simulink model "final_hybrid_system_load_variation"  (R2018a)
settings: Solver=ode23tb  StartTime=0.0  StopTime=4  FixedStep=1e-6  RelTol=1e-3
values from neighbouring files (symbols this model uses):
  Dp = 636    [sychrocovnverter.m]
  Dq = 100/155.35    (= 0.643707756678)    [sychrocovnverter.m]
  J = 2    [sychrocovnverter.m]
  K = 500    [sychrocovnverter.m]
  p = 1    [sychrocovnverter.m]
  Ts = 1e-6    (= 1e-06)    [sychrocovnverter.m]
  w_n = 2*pi*50    (= 314.159265359)    [sychrocovnverter.m]
  w_ref = w_n    (= 314.159265359)    [sychrocovnverter.m]
undefined symbols (not defined in the file or in its folder): sigbuilder_block
libraries: powerlib x73, powerlib_meascontrol x12, simulink x3, sps_avr x1, spsHTGModel x1, re_lib x1
settings Model: SimulationMode=accelerator  Creator=deep  LastModifiedBy=Electrical
settings SolverCC: AlgebraicLoopSolver=LineSearch
settings OptimizationCC: EfficientMapNaN2IntZero=off
settings HardwareCC: TargetBitPerPointer=64  TargetBitPerSizeT=64  TargetBitPerPtrDiffT=64  TargetLongLongMode=on  TargetIntDivRoundTo=Zero  TargetEndianess=LittleEndian  TargetWordSize=64  TargetHWDeviceType=MATLAB Host  ProdEqTarget=off
settings SFSimCC: SimUseLocalCustomCode=on
settings RTWCC: RTWUseLocalCustomCode=on
settings CodeAppCC: MaxIdLength=128
settings GRTTargetCC: TargetLangStandard=C89/C90 (ANSI)  CombineOutputUpdateFcns=off  GRTInterface=on

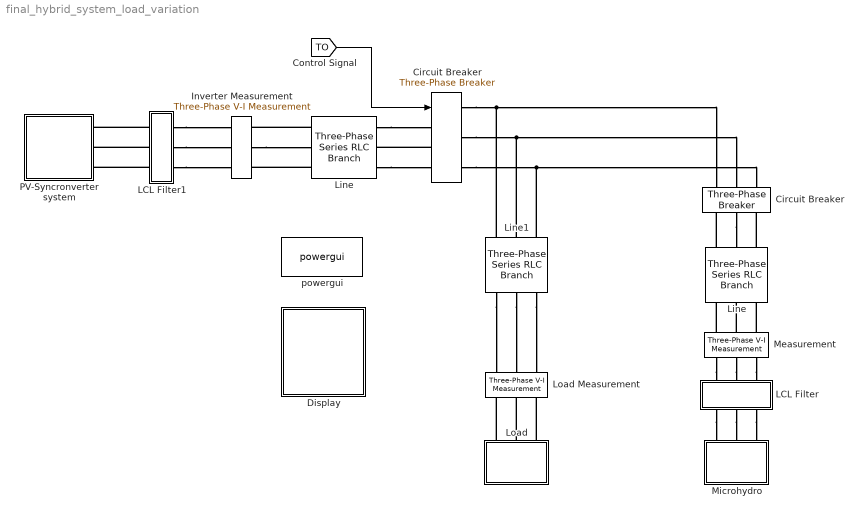
== system final_hybrid_system_load_variation ==
  Circuit Breaker : powerlib/Elements/Three-Phase Breaker  InitialState=open  SwitchA=on  SwitchB=on  SwitchC=on  SwitchTimes=[0.5 4]  External=off  BreakerResistance=0.00001  SnubberResistance=500000  SnubberCapacitance=inf  Measurements=None
  "Circuit Breaker  " : powerlib/Elements/Three-Phase Breaker  InitialState=closed  SwitchA=on  SwitchB=on  SwitchC=on  SwitchTimes=[0.5 4]  External=on  BreakerResistance=0.00001  SnubberResistance=500000  SnubberCapacitance=inf  Measurements=None
  Display : Subsystem
  Inverter Measurement : powerlib/Measurements/Three-Phase V-I Measurement  VoltageMeasurement=phase-to-ground  SetLabelV=on  LabelV=Vinv  Vpu=off  VpuLL=off  CurrentMeasurement=yes  SetLabelI=on  LabelI=Iinv  Ipu=off  Pbase=100e6  Vbase=500e3  OutputType=Complex  PhasorSimulation=off  PSBequivalent=0
  LCL Filter : Subsystem  mask{L=0.5e-3, C=100e-6}
      mask prompts: L "Inductance(L)"; C "Capacitance(C)"
  LCL Filter1 : Subsystem  mask{L=10e-3, C=0.5e-6}
      mask prompts: L "Inductance(L)"; C "Capacitance(C)"
  Line : powerlib/Elements/Three-Phase Series RLC Branch  LConnTagsString=A|B|C  RConnTagsString=A|B|C  BranchType=RL  Resistance=0.1  Inductance=0.0125  Capacitance=0  Measurements=None
  "Line  " : powerlib/Elements/Three-Phase Series RLC Branch  LConnTagsString=A|B|C  RConnTagsString=A|B|C  BranchType=RL  Resistance=0.1  Inductance=0.0125  Capacitance=0  Measurements=None
  Line1 : powerlib/Elements/Three-Phase Series RLC Branch  LConnTagsString=A|B|C  RConnTagsString=A|B|C  BranchType=RL  Resistance=0.1  Inductance=0.005  Capacitance=0  Measurements=None
  Load : Subsystem
  Load Measurement : powerlib/Measurements/Three-Phase V-I Measurement  VoltageMeasurement=phase-to-ground  SetLabelV=on  LabelV=Vload  Vpu=off  VpuLL=off  CurrentMeasurement=yes  SetLabelI=on  LabelI=Iload  Ipu=off  Pbase=100e6  Vbase=500e3  OutputType=Complex  PhasorSimulation=off  PSBequivalent=0
  Measurement : powerlib/Measurements/Three-Phase V-I Measurement  VoltageMeasurement=phase-to-ground  SetLabelV=on  LabelV=Vgrid  Vpu=off  VpuLL=off  CurrentMeasurement=yes  SetLabelI=on  LabelI=Igrid  Ipu=off  Pbase=100e6  Vbase=500e3  OutputType=Complex  PhasorSimulation=off  PSBequivalent=0
  Microhydro : Subsystem
  PV-Syncronverter system : Subsystem
  powergui : powerlib/powergui  Priority=1  SimulationMode=Discrete  SampleTime=1e-6  frequency=60  Iterations=50  frequencyindice=0  Pbase=100e6  ErrMax=1e-4  UnitsV=kV  UnitsW=MW  buscounter=0  FunctionMessages=off  echomessages=off  EnableUseOfTLC=off  CurrentSourceSwitches=off  DisableSnubberDevices=off  DisableRonSwitches=off  DisableVfSwitches=off  DisplayEquations=off  SolverType=Tustin/Backward Euler (TBE)  Interpol=off  ExternalGateDelay=off  methode=off  Ts=100  x0status=zero  SPID=off  SwTol=0  HookPort=off  RestoreLinks=warning  ResistiveCurrentMeasurement=off  Frange=[0:2:500]  Ylog=off  Xlog=on  ShowGrid=off  save=off  variable=ZData  structure=logsout  ZoomFFT=off  StartTime=0.0  cycles=1  DisplayStyle=1  fundamental=60  FreqAxis=off  MaxFrequency=1000  frequencyindicesteady=1  RmsSteady=1  display=off
  wires:
  [TO] -> "Circuit Breaker  "/1
  connections:
  "Circuit Breaker  "/RConn1 -- Circuit Breaker/RConn1 -- Line1/LConn1
  "Circuit Breaker  "/RConn3 -- Circuit Breaker/RConn3 -- Line1/LConn3
  LCL Filter/LConn2 -- Microhydro/RConn2
  LCL Filter/LConn3 -- Microhydro/RConn3
  LCL Filter/LConn1 -- Microhydro/RConn1
  "Circuit Breaker  "/RConn2 -- Circuit Breaker/RConn2 -- Line1/LConn2
  Line/RConn1 -- Circuit Breaker/LConn1
  Circuit Breaker/LConn2 -- Line/RConn2
  Line/RConn3 -- Circuit Breaker/LConn3
  Measurement/RConn1 -- Line/LConn1
  Measurement/RConn2 -- Line/LConn2
  Measurement/RConn3 -- Line/LConn3
  Measurement/LConn1 -- LCL Filter/RConn1
  Measurement/LConn2 -- LCL Filter/RConn2
  Measurement/LConn3 -- LCL Filter/RConn3
  Load/LConn1 -- Load Measurement/RConn1
  Load/LConn2 -- Load Measurement/RConn2
  Load/LConn3 -- Load Measurement/RConn3
  "Line  "/RConn1 -- "Circuit Breaker  "/LConn1
  "Circuit Breaker  "/LConn2 -- "Line  "/RConn2
  "Line  "/RConn3 -- "Circuit Breaker  "/LConn3
  "Line  "/LConn1 -- Inverter Measurement/RConn1
  Inverter Measurement/RConn2 -- "Line  "/LConn2
  "Line  "/LConn3 -- Inverter Measurement/RConn3
  LCL Filter1/LConn1 -- PV-Syncronverter system/RConn1
  LCL Filter1/LConn2 -- PV-Syncronverter system/RConn2
  LCL Filter1/LConn3 -- PV-Syncronverter system/RConn3
  LCL Filter1/RConn1 -- Inverter Measurement/LConn1
  LCL Filter1/RConn2 -- Inverter Measurement/LConn2
  LCL Filter1/RConn3 -- Inverter Measurement/LConn3
  Line1/RConn1 -- Load Measurement/LConn1
  Line1/RConn2 -- Load Measurement/LConn2
  Line1/RConn3 -- Load Measurement/LConn3

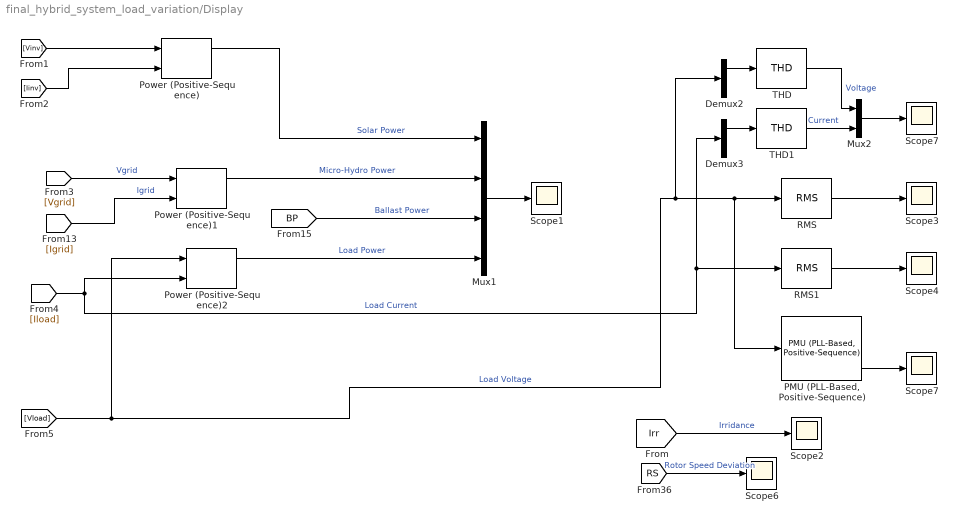
== system final_hybrid_system_load_variation/Display ==
  Demux2 : Demux  Outputs=3
  Demux3 : Demux  Outputs=3
  Mux1 : Mux
  Mux2 : Mux  Inputs=2
  "PMU (PLL-Based, Positive-Sequence)" : powerlib_meascontrol/Measurements/PMU (PLL-Based, Positive-Sequence)  nominalFrequency=50  samplingRate=64  reportingFactor=1
      settings: SourceProductName=Simscape Power Systems  SourceProductBaseCode=PS
  Power (Positive-Sequence) : powerlib_meascontrol/Measurements/Power (Positive-Sequence)  Freq=50  Vinit=[0, 0]  Iinit=[0, 0]  Ts=0
      settings: SourceProductName=Simscape Power Systems  SourceProductBaseCode=PS
  Power (Positive-Sequence)1 : powerlib_meascontrol/Measurements/Power (Positive-Sequence)  Freq=50  Vinit=[0, 0]  Iinit=[0, 0]  Ts=0
      settings: SourceProductName=Simscape Power Systems  SourceProductBaseCode=PS
  Power (Positive-Sequence)2 : powerlib_meascontrol/Measurements/Power (Positive-Sequence)  Freq=50  Vinit=[0, 0]  Iinit=[0, 0]  Ts=0
      settings: SourceProductName=Simscape Power Systems  SourceProductBaseCode=PS
  RMS : powerlib_meascontrol/Measurements/RMS  TrueRMS=on  Freq=50  RMSInit=0  Ts=0
  RMS1 : powerlib_meascontrol/Measurements/RMS  TrueRMS=on  Freq=50  RMSInit=0  Ts=0
  Scope{1..4,6..7} (6 alike) : Scope
  "Scope7 " : Scope
  THD : powerlib_meascontrol/Measurements/THD  Freq=50  Ts=0
  THD1 : powerlib_meascontrol/Measurements/THD  Freq=50  Ts=0
  wires:
  [Iinv] -> Power (Positive-Sequence)/2
  [Vinv] -> Power (Positive-Sequence)/1
  Power (Positive-Sequence)/1 -> Mux1/1  "Solar Power"
  [Igrid] -> Power (Positive-Sequence)1/2  "Igrid"
  [Vgrid] -> Power (Positive-Sequence)1/1  "Vgrid"
  [Iload] -> RMS1/1, Demux3/1, Power (Positive-Sequence)2/2  "Load Current"
  [Irr] -> Scope2/1  "Irridance"
  [RS] -> Scope6/1  "Rotor Speed Deviation"
  [Vload] -> Power (Positive-Sequence)2/1, Demux2/1, "PMU (PLL-Based, Positive-Sequence)"/1, RMS/1  "Load Voltage"
  Mux1/1 -> Scope1/1
  Power (Positive-Sequence)1/1 -> Mux1/2  "Micro-Hydro Power"
  [BP] -> Mux1/3  "Ballast Power"
  RMS/1 -> Scope3/1
  RMS1/1 -> Scope4/1
  "PMU (PLL-Based, Positive-Sequence)"/3 -> Scope7/1
  Demux2/1 -> THD/1
  Demux3/1 -> THD1/1
  THD/1 -> Mux2/1  "Voltage"
  THD1/1 -> Mux2/2  "Current"
  Mux2/1 -> "Scope7 "/1
  Power (Positive-Sequence)2/1 -> Mux1/4  "Load Power"

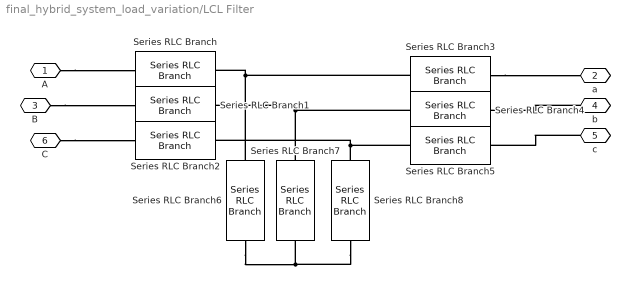
== system final_hybrid_system_load_variation/LCL Filter ==
  Series RLC Branch{,1..5} (6 alike) : powerlib/Elements/Series RLC Branch  LConnTagsString=__new0  RConnTagsString=__new0  BranchType=L  Resistance=1  Inductance=L  SetiL0=off  InitialCurrent=0  Capacitance=1e-6  Setx0=off  InitialVoltage=0  Measurements=None
  Series RLC Branch6 : powerlib/Elements/Series RLC Branch  LConnTagsString=__new0  RConnTagsString=__new0  BranchType=C  Resistance=1  Inductance=0.5e-3  SetiL0=off  InitialCurrent=0  Capacitance=C  Setx0=off  InitialVoltage=0  Measurements=None
  Series RLC Branch7 : powerlib/Elements/Series RLC Branch  LConnTagsString=__new0  RConnTagsString=__new0  BranchType=C  Resistance=1  Inductance=0.5e-3  SetiL0=off  InitialCurrent=0  Capacitance=C  Setx0=off  InitialVoltage=0  Measurements=None
  Series RLC Branch8 : powerlib/Elements/Series RLC Branch  LConnTagsString=__new0  RConnTagsString=__new0  BranchType=C  Resistance=1  Inductance=0.5e-3  SetiL0=off  InitialCurrent=0  Capacitance=C  Setx0=off  InitialVoltage=0  Measurements=None
  A : PMIOPort  Side=Left
  a : PMIOPort  Port=2  Side=Right
  B : PMIOPort  Port=3  Side=Left
  b : PMIOPort  Port=4  Side=Right
  c : PMIOPort  Port=5  Side=Right
  C : PMIOPort  Port=6  Side=Left
  connections:
  C/RConn1 -- Series RLC Branch2/LConn1
  Series RLC Branch3/LConn1 -- Series RLC Branch/RConn1 -- Series RLC Branch6/LConn1
  Series RLC Branch3/RConn1 -- a/RConn1
  Series RLC Branch6/RConn1 -- Series RLC Branch8/RConn1 -- Series RLC Branch7/RConn1
  Series RLC Branch5/LConn1 -- Series RLC Branch2/RConn1 -- Series RLC Branch8/LConn1
  Series RLC Branch4/LConn1 -- Series RLC Branch1/RConn1 -- Series RLC Branch7/LConn1
  c/RConn1 -- Series RLC Branch5/RConn1
  A/RConn1 -- Series RLC Branch/LConn1
  B/RConn1 -- Series RLC Branch1/LConn1
  b/RConn1 -- Series RLC Branch4/RConn1

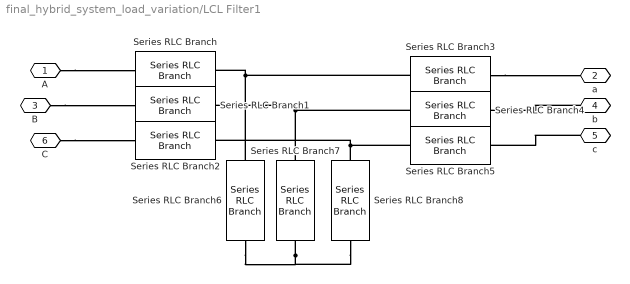
== system final_hybrid_system_load_variation/LCL Filter1 ==
  Series RLC Branch{,1..5} (6 alike) : powerlib/Elements/Series RLC Branch  LConnTagsString=__new0  RConnTagsString=__new0  BranchType=L  Resistance=1  Inductance=L  SetiL0=off  InitialCurrent=0  Capacitance=1e-6  Setx0=off  InitialVoltage=0  Measurements=None
  Series RLC Branch6 : powerlib/Elements/Series RLC Branch  LConnTagsString=__new0  RConnTagsString=__new0  BranchType=C  Resistance=1  Inductance=0.5e-3  SetiL0=off  InitialCurrent=0  Capacitance=C  Setx0=off  InitialVoltage=0  Measurements=None
  Series RLC Branch7 : powerlib/Elements/Series RLC Branch  LConnTagsString=__new0  RConnTagsString=__new0  BranchType=C  Resistance=1  Inductance=0.5e-3  SetiL0=off  InitialCurrent=0  Capacitance=C  Setx0=off  InitialVoltage=0  Measurements=None
  Series RLC Branch8 : powerlib/Elements/Series RLC Branch  LConnTagsString=__new0  RConnTagsString=__new0  BranchType=C  Resistance=1  Inductance=0.5e-3  SetiL0=off  InitialCurrent=0  Capacitance=C  Setx0=off  InitialVoltage=0  Measurements=None
  A : PMIOPort  Side=Left
  a : PMIOPort  Port=2  Side=Right
  B : PMIOPort  Port=3  Side=Left
  b : PMIOPort  Port=4  Side=Right
  c : PMIOPort  Port=5  Side=Right
  C : PMIOPort  Port=6  Side=Left
  connections:
  b/RConn1 -- Series RLC Branch4/RConn1
  B/RConn1 -- Series RLC Branch1/LConn1
  A/RConn1 -- Series RLC Branch/LConn1
  c/RConn1 -- Series RLC Branch5/RConn1
  Series RLC Branch7/LConn1 -- Series RLC Branch1/RConn1 -- Series RLC Branch4/LConn1
  Series RLC Branch8/LConn1 -- Series RLC Branch2/RConn1 -- Series RLC Branch5/LConn1
  Series RLC Branch7/RConn1 -- Series RLC Branch8/RConn1 -- Series RLC Branch6/RConn1
  Series RLC Branch3/RConn1 -- a/RConn1
  Series RLC Branch6/LConn1 -- Series RLC Branch/RConn1 -- Series RLC Branch3/LConn1
  C/RConn1 -- Series RLC Branch2/LConn1

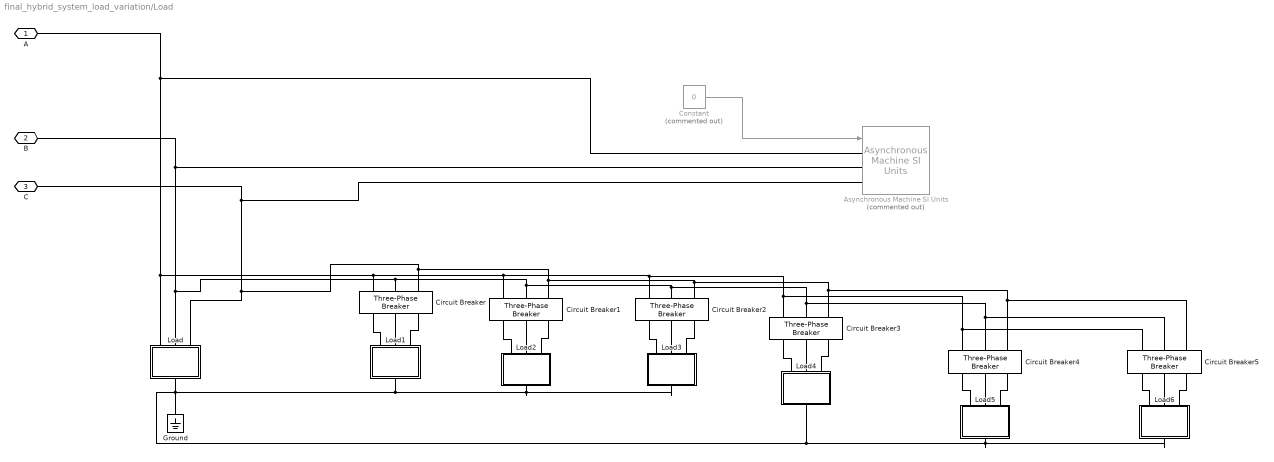
== system final_hybrid_system_load_variation/Load ==
  Asynchronous Machine SI Units : powerlib/Machines/Asynchronous Machine SI Units  Commented=on  RotorType=Squirrel-cage  PresetModel="15:  5.4 HP (4KW)   400 V  50Hz 1430 RPM"  MechanicalLoad=Torque Tm  ShowDetailedParameters=on  ReferenceFrame=Rotor  Units=SI  MeasurementBus=off  NominalParameters=[4000 400 50]  Stator=[1.405 0.005839]  Rotor=[1.395 0.005839]  Cage1=[0.4155 0.002066]  Cage2=[0.4168 0.0003495]  Lm=0.1722  Mechanical=[0.0131 0.002985 2]  PolePairs=2  InitialConditions=[0 0 0 0 0 0 0 0]  SimulateSaturation=off  Saturation=[14.03593122, 27.81365428, 53.79336849, 72.68890987, 97.98006896, 148.6815601, 215.7428561, 302.9841135, 428.7778367 ; 230, 322, 414, 460, 506, 552, 598, 644, 690]  LoadFlowParameters=1492000  TsPowergui=0  TsBlock=-1  IterativeModel=Trapezoidal non iterative  IterativeDiscreteModel=Trapezoidal non iterative  Pmec=1.492e+006
  Circuit Breaker : powerlib/Elements/Three-Phase Breaker  InitialState=open  SwitchA=on  SwitchB=on  SwitchC=on  SwitchTimes=[1 4]  External=off  BreakerResistance=0.00001  SnubberResistance=500000  SnubberCapacitance=inf  Measurements=None
  Circuit Breaker1 : powerlib/Elements/Three-Phase Breaker  InitialState=open  SwitchA=on  SwitchB=on  SwitchC=on  SwitchTimes=[1.5 4]  External=off  BreakerResistance=0.00001  SnubberResistance=500000  SnubberCapacitance=inf  Measurements=None
  Circuit Breaker2 : powerlib/Elements/Three-Phase Breaker  InitialState=open  SwitchA=on  SwitchB=on  SwitchC=on  SwitchTimes=[2 4]  External=off  BreakerResistance=0.00001  SnubberResistance=500000  SnubberCapacitance=inf  Measurements=None
  Circuit Breaker3 : powerlib/Elements/Three-Phase Breaker  InitialState=open  SwitchA=on  SwitchB=on  SwitchC=on  SwitchTimes=[2.5 4]  External=off  BreakerResistance=0.00001  SnubberResistance=500000  SnubberCapacitance=inf  Measurements=None
  Circuit Breaker4 : powerlib/Elements/Three-Phase Breaker  InitialState=open  SwitchA=on  SwitchB=on  SwitchC=on  SwitchTimes=[3 4]  External=off  BreakerResistance=0.00001  SnubberResistance=500000  SnubberCapacitance=inf  Measurements=None
  Circuit Breaker5 : powerlib/Elements/Three-Phase Breaker  InitialState=open  SwitchA=on  SwitchB=on  SwitchC=on  SwitchTimes=[3.5 4]  External=off  BreakerResistance=0.00001  SnubberResistance=500000  SnubberCapacitance=inf  Measurements=None
  Constant : Constant  Commented=on  Value=0
  Ground : powerlib/Elements/Ground  LConnTagsString=a
  Load : Subsystem  mask{R=50}
      mask prompts: R "Load Resistance"
      mask DialogControl DescTextVar Prompt: Load in terms of Resistance
  Load1 : Subsystem  mask{R=80}
      mask prompts: R "Load Resistance"
      mask DialogControl DescTextVar Prompt: Load in terms of Resistance
  Load2 : Subsystem  mask{R=80}
      mask prompts: R "Load Resistance"
      mask DialogControl DescTextVar Prompt: Load in terms of Resistance
  Load3 : Subsystem  mask{R=80}
      mask prompts: R "Load Resistance"
      mask DialogControl DescTextVar Prompt: Load in terms of Resistance
  Load4 : Subsystem  mask{R=80}
      mask prompts: R "Load Resistance"
      mask DialogControl DescTextVar Prompt: Load in terms of Resistance
  Load5 : Subsystem  mask{R=80}
      mask prompts: R "Load Resistance"
      mask DialogControl DescTextVar Prompt: Load in terms of Resistance
  Load6 : Subsystem  mask{R=80}
      mask prompts: R "Load Resistance"
      mask DialogControl DescTextVar Prompt: Load in terms of Resistance
  A : PMIOPort  Side=Left
  B : PMIOPort  Port=2  Side=Left
  C : PMIOPort  Port=3  Side=Left
  wires:
  Constant/1 -> Asynchronous Machine SI Units/1
  connections:
  Ground/LConn1 -- Load6/RConn1 -- Load5/RConn1 -- Load4/RConn1 -- Load3/RConn1 -- Load2/RConn1 -- Load1/RConn1 -- Load/RConn1
  Load/LConn1 -- Circuit Breaker5/RConn1 -- Circuit Breaker4/RConn1 -- Circuit Breaker3/RConn1 -- Circuit Breaker2/RConn1 -- Circuit Breaker1/RConn1 -- Circuit Breaker/RConn1 -- Asynchronous Machine SI Units/LConn1 -- A/RConn1
  Load/LConn2 -- Circuit Breaker5/RConn2 -- Circuit Breaker4/RConn2 -- Circuit Breaker3/RConn2 -- Circuit Breaker2/RConn2 -- Circuit Breaker1/RConn2 -- Circuit Breaker/RConn2 -- B/RConn1 -- Asynchronous Machine SI Units/LConn2
  Load/LConn3 -- Circuit Breaker5/RConn3 -- Circuit Breaker4/RConn3 -- Circuit Breaker3/RConn3 -- Circuit Breaker2/RConn3 -- Circuit Breaker1/RConn3 -- Circuit Breaker/RConn3 -- Asynchronous Machine SI Units/LConn3 -- C/RConn1
  Circuit Breaker/LConn2 -- Load1/LConn2
  Circuit Breaker/LConn1 -- Load1/LConn1
  Circuit Breaker/LConn3 -- Load1/LConn3
  Circuit Breaker1/LConn2 -- Load2/LConn2
  Circuit Breaker1/LConn1 -- Load2/LConn1
  Circuit Breaker1/LConn3 -- Load2/LConn3
  Circuit Breaker2/LConn2 -- Load3/LConn2
  Circuit Breaker2/LConn1 -- Load3/LConn1
  Circuit Breaker2/LConn3 -- Load3/LConn3
  Circuit Breaker3/LConn1 -- Load4/LConn1
  Circuit Breaker3/LConn3 -- Load4/LConn3
  Circuit Breaker3/LConn2 -- Load4/LConn2
  Load5/LConn1 -- Circuit Breaker4/LConn1
  Circuit Breaker4/LConn2 -- Load5/LConn2
  Load5/LConn3 -- Circuit Breaker4/LConn3
  Circuit Breaker5/LConn2 -- Load6/LConn2
  Load6/LConn1 -- Circuit Breaker5/LConn1
  Load6/LConn3 -- Circuit Breaker5/LConn3

== system final_hybrid_system_load_variation/Microhydro ==
  Bus Selector : BusSelector  OutputSignals="Mechanical.Rotor speed deviation  dw (pu),dq0 components.Stator voltage  vd (pu),dq0 components.Stator voltage  vq (pu)"
  Electronic Load Controller : Subsystem
  Excitation System (IEEE Type I) : sps_avr/Excitation System  tr=20e-3  reg=[ 300, 0.001 ]  exc=[ 1, 0 ]  tgr=[ 0, 0 ]  damp=[ 0.001, 0.1 ]  sat=[ 0, 0 ]  lim=[ -11.5, 11.5, 0 ]  v0="[1.0  1.28]"
      settings: SourceProductName=Simscape Power Systems  SourceProductBaseCode=PS
  Ground : Ground
  Parasitic Load (400 W) : powerlib/Elements/Three-Phase Series RLC Load  LConnTagsString=A|B|C  Configuration=Y (grounded)  NominalVoltage=400  Vabc=[1e3 1e3 1e3]  Vabcp=[1e3 1e3 1e3]  NominalFrequency=50  UnbalancedPower=off  ActivePower=400  InductivePower=0  CapacitivePower=0  Pabc=[10e3 9e3 11e3]  QLabc=[100 90 110]  QCabc=[100 90 110]  Pabcp=[10e3 9e3 11e3]  QLabcp=[100 90 110]  QCabcp=[100 90 110]  Measurements=None  LoadType=constant Z
  Pm(pu) : Constant  SampleTime=-1
  "Synchronous Machine (8.1kVA, 1500RPM, 50Hz)" : powerlib/Machines/Synchronous Machine pu Fundamental  PresetModel=01: 50Hz 400V 8.1kVA 1500RPM  MechanicalLoad=Mechanical power Pm  ShowDetailedParameters=on  RotorType=Salient-pole  Units=per unit fundamental parameters  MeasurementBus=off  NominalParameters=[8100 400 50]  Stator=[0.08201 0.072 1.728 0.823]  Field=[0.06117 0.1801]  Dampers2=[0.0652, 0.5134, 0.0287, 0.2553, 7.765e-3, 0.9167 ]  Dampers1=[0.1591 0.1166 0.2416 0.1615]  Mechanical=[0.1406 0.02742 2]  PolePairs=2  InitialConditions="[ 0  0  0  0  0  0  -120  -240  1 ]"  SetSaturation=off  Saturation=[0.6404,0.7127,0.8441,0.9214,0.9956,1.082,1.19,1.316,1.457;0.7,0.7698,0.8872,0.9466,0.9969,1.046,1.1,1.151,1.201]  LoadFlowParameters=[1,0,0,0,0]  TsPowergui=0  TsBlock=-1  IterativeModel=Trapezoidal non iterative  IterativeDiscreteModel=Trapezoidal non iterative  BusType=PV  Pref=8100  Qref=0  Qmin=-inf  Qmax=inf  PLF=0  QLF=0
      settings: SourceProductName=Simscape Power Systems  SourceProductBaseCode=PS
  Vref(pu) : Constant  Value=1.02  SampleTime=-1
  turbine : spsHTGModel/Discrete/turbine  SystemSampleTime=-1
      link override Gain2: Gain=1/1
      link override beta: Gain=1
      link override position: InitialCondition=1
      link override turbine gain: Gain=1
  A : PMIOPort  Side=Right
  B : PMIOPort  Port=2  Side=Right
  C : PMIOPort  Port=3  Side=Right
  wires:
  Bus Selector/1 -> turbine/1, Electronic Load Controller/1(Rotor Speed(pu))  "<Rotor speed deviation  dw (pu)>"
  "Synchronous Machine (8.1kVA, 1500RPM, 50Hz)"/1 -> Bus Selector/1
  Excitation System (IEEE Type I)/1 -> "Synchronous Machine (8.1kVA, 1500RPM, 50Hz)"/2
  Bus Selector/2 -> Excitation System (IEEE Type I)/2  "<Stator voltage  vd (pu)>"
  Bus Selector/3 -> Excitation System (IEEE Type I)/3  "<Stator voltage  vq (pu)>"
  Ground/1 -> Excitation System (IEEE Type I)/4
  Pm(pu)/1 -> turbine/2
  turbine/1 -> "Synchronous Machine (8.1kVA, 1500RPM, 50Hz)"/1
  Vref(pu)/1 -> Excitation System (IEEE Type I)/1
  connections:
  Electronic Load Controller/LConn2 -- B/RConn1 -- Parasitic Load (400 W)/LConn2 -- "Synchronous Machine (8.1kVA, 1500RPM, 50Hz)"/RConn2
  Electronic Load Controller/LConn1 -- A/RConn1 -- Parasitic Load (400 W)/LConn1 -- "Synchronous Machine (8.1kVA, 1500RPM, 50Hz)"/RConn1
  Electronic Load Controller/LConn3 -- Parasitic Load (400 W)/LConn3 -- C/RConn1 -- "Synchronous Machine (8.1kVA, 1500RPM, 50Hz)"/RConn3

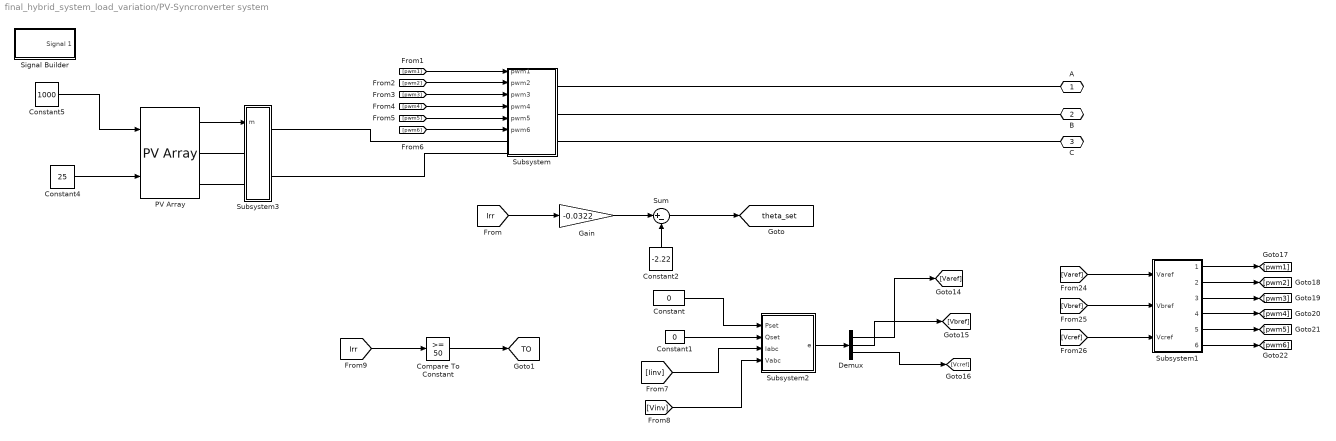
== system final_hybrid_system_load_variation/PV-Syncronverter system ==
  Compare To Constant : simulink/Logic and Bit Operations/Compare To Constant  relop=>=  const=50  OutDataTypeStr=boolean
  Constant : Constant  Value=0
  Constant1 : Constant  Value=0
  Constant2 : Constant  Value=-2.22
  Constant4 : Constant  Value=25
  Constant5 : Constant  Value=1000
  Demux : Demux  Outputs=3
  Gain : Gain  Gain=-0.0322
  PV Array : re_lib/Solar/PV Array  Npar=2  Nser=25  PlotType=array @ 25 deg.C & specified irradiances  S_vec="[ 150 120  100 ]"  Temp_C_vec="[ 45 25  ]"  ModuleName=1Soltech 1STH-215-P  PlotWhenSelected=off  Pm=213.15  Ncell=60  Voc=36.3  Isc=7.84  Vm=29  Im=7.35  beta_Voc_pc=-0.36099  alpha_Isc_pc=0.102  beta_Voc=-0.13104  alpha_Isc=0.007997  IL=7.8649  I0=2.9259e-10  nI=0.98117  Rsh=313.3991  Rs=0.39383  BAL=on  Tc=1e-6  Tfilter=1e-6
  Signal Builder : Subsystem  Tag=STV Subsys  LoadFcn=sigbuilder_block('load');  StartFcn=sigbuilder_block('start');  StopFcn=sigbuilder_block('stop');  ClipboardFcn=sigbuilder_block('clipboard');  mask(Sigbuilder block){tuvar=[0:10]}
      mask help: Simulink:masks:SigbuilderBlock_MD
      mask init:
      | if ~strcmp(get_param(bdroot(gcbh),'SimulationStatus'),'stopped') tuvar = sigbuilder_block('maskInit'); end
      settings: CopyFcn=sigbuilder_block('copy');  DeleteFcn=sigbuilder_block('delete');  ModelCloseFcn=sigbuilder_block('modelClose');  PreSaveFcn=sigbuilder_block('preSave');  PauseFcn=sigbuilder_block('pause');  ContinueFcn=sigbuilder_block('continue');  NameChangeFcn=sigbuilder_block('namechange');  OpenFcn=sigbuilder_block('open',[6 0 1012.5 424.5 ]);  CloseFcn=sigbuilder_block('close');
      mask Display: plot(0, 0, 100, 100,[2, 2, 32, 32, 2], [68, 8, 8, 68, 68],[32, 2], [38, 38], [32, 19, 2],[53, 60, 44], [32, 17, 17, 2],[16, 16, 31, 31]);txt = getActiveGroup(gcbh);text(2, 100, txt,'verticalAlignment', 'top');
  Subsystem : Subsystem
  Subsystem1 : Subsystem
  Subsystem2 : Subsystem
  Subsystem3 : Subsystem
  Sum : Sum  Inputs=|+-
  A : PMIOPort  Side=Right
  B : PMIOPort  Port=2  Side=Right
  C : PMIOPort  Port=3  Side=Right
  tag scope: TO=global, theta_set=global
  wires:
  [pwm4] -> Subsystem/4(pwm4)
  Subsystem1/4(pwm4) -> [pwm4]
  [pwm5] -> Subsystem/5(pwm5)
  [pwm6] -> Subsystem/6(pwm6)
  Subsystem1/5(pwm5) -> [pwm5]
  [pwm2] -> Subsystem/2(pwm2)
  [Vbref] -> Subsystem1/2(Vbref)
  Subsystem1/2(pwm2) -> [pwm2]
  Subsystem1/1(pwm1) -> [pwm1]
  [pwm3] -> Subsystem/3(pwm3)
  Subsystem1/3(pwm3) -> [pwm3]
  [Vcref] -> Subsystem1/3(Vcref)
  [Varef] -> Subsystem1/1("Varef ")
  Subsystem1/6(pwm6) -> [pwm6]
  [pwm1] -> Subsystem/1(pwm1)
  [Iinv] -> Subsystem2/3("Iabc ")
  Subsystem2/1(e) -> Demux/1
  Demux/1 -> [Varef]
  Demux/2 -> [Vbref]
  Demux/3 -> [Vcref]
  Constant/1 -> Subsystem2/1("Pset ")
  Constant1/1 -> Subsystem2/2(Qset)
  [Vinv] -> Subsystem2/4(Vabc)
  Constant4/1 -> PV Array/2
  PV Array/1 -> Subsystem3/1(m)
  [Irr] -> Compare To Constant/1
  Compare To Constant/1 -> [TO]
  [Irr] -> Gain/1
  Constant2/1 -> Sum/2
  Gain/1 -> Sum/1
  Sum/1 -> [theta_set]
  Constant5/1 -> PV Array/1
  connections:
  Subsystem/RConn3 -- C/RConn1
  Subsystem/RConn2 -- B/RConn1
  Subsystem/RConn1 -- A/RConn1
  Subsystem3/RConn1 -- Subsystem/LConn1
  Subsystem3/RConn2 -- Subsystem/LConn2
  PV Array/RConn1 -- Subsystem3/LConn1
  PV Array/RConn2 -- Subsystem3/LConn2

== system final_hybrid_system_load_variation/Load/Load ==
  1 : powerlib/Elements/Series RLC Branch  LConnTagsString=__new0  RConnTagsString=__new0  BranchType=R  Resistance=R  Inductance=10e-3  SetiL0=off  InitialCurrent=0  Capacitance=1e-6  Setx0=off  InitialVoltage=0  Measurements=None
  2 : powerlib/Elements/Series RLC Branch  LConnTagsString=__new0  RConnTagsString=__new0  BranchType=R  Resistance=R  Inductance=10e-3  SetiL0=off  InitialCurrent=0  Capacitance=1e-6  Setx0=off  InitialVoltage=0  Measurements=None
  3 : powerlib/Elements/Series RLC Branch  LConnTagsString=__new0  RConnTagsString=__new0  BranchType=R  Resistance=R  Inductance=10e-3  SetiL0=off  InitialCurrent=0  Capacitance=1e-6  Setx0=off  InitialVoltage=0  Measurements=None
  A : PMIOPort  Side=Left
  B : PMIOPort  Port=2  Side=Left
  C : PMIOPort  Port=3  Side=Left
  N : PMIOPort  Port=4  Side=Right
  connections:
  A/RConn1 -- 2/LConn1
  B/RConn1 -- 1/LConn1
  C/RConn1 -- 3/LConn1
  1/RConn1 -- 3/RConn1 -- N/RConn1 -- 2/RConn1

== system final_hybrid_system_load_variation/Load/Load1 ==
  1 : powerlib/Elements/Series RLC Branch  LConnTagsString=__new0  RConnTagsString=__new0  BranchType=R  Resistance=R  Inductance=10e-3  SetiL0=off  InitialCurrent=0  Capacitance=1e-6  Setx0=off  InitialVoltage=0  Measurements=None
  2 : powerlib/Elements/Series RLC Branch  LConnTagsString=__new0  RConnTagsString=__new0  BranchType=R  Resistance=R  Inductance=10e-3  SetiL0=off  InitialCurrent=0  Capacitance=1e-6  Setx0=off  InitialVoltage=0  Measurements=None
  3 : powerlib/Elements/Series RLC Branch  LConnTagsString=__new0  RConnTagsString=__new0  BranchType=R  Resistance=R  Inductance=10e-3  SetiL0=off  InitialCurrent=0  Capacitance=1e-6  Setx0=off  InitialVoltage=0  Measurements=None
  A : PMIOPort  Side=Left
  B : PMIOPort  Port=2  Side=Left
  C : PMIOPort  Port=3  Side=Left
  N : PMIOPort  Port=4  Side=Right
  connections:
  A/RConn1 -- 2/LConn1
  B/RConn1 -- 1/LConn1
  C/RConn1 -- 3/LConn1
  1/RConn1 -- 3/RConn1 -- N/RConn1 -- 2/RConn1

== system final_hybrid_system_load_variation/Load/Load2 ==
  1 : powerlib/Elements/Series RLC Branch  LConnTagsString=__new0  RConnTagsString=__new0  BranchType=R  Resistance=R  Inductance=10e-3  SetiL0=off  InitialCurrent=0  Capacitance=1e-6  Setx0=off  InitialVoltage=0  Measurements=None
  2 : powerlib/Elements/Series RLC Branch  LConnTagsString=__new0  RConnTagsString=__new0  BranchType=R  Resistance=R  Inductance=10e-3  SetiL0=off  InitialCurrent=0  Capacitance=1e-6  Setx0=off  InitialVoltage=0  Measurements=None
  3 : powerlib/Elements/Series RLC Branch  LConnTagsString=__new0  RConnTagsString=__new0  BranchType=R  Resistance=R  Inductance=10e-3  SetiL0=off  InitialCurrent=0  Capacitance=1e-6  Setx0=off  InitialVoltage=0  Measurements=None
  A : PMIOPort  Side=Left
  B : PMIOPort  Port=2  Side=Left
  C : PMIOPort  Port=3  Side=Left
  N : PMIOPort  Port=4  Side=Right
  connections:
  A/RConn1 -- 2/LConn1
  B/RConn1 -- 1/LConn1
  C/RConn1 -- 3/LConn1
  1/RConn1 -- 3/RConn1 -- N/RConn1 -- 2/RConn1

== system final_hybrid_system_load_variation/Load/Load3 ==
  1 : powerlib/Elements/Series RLC Branch  LConnTagsString=__new0  RConnTagsString=__new0  BranchType=R  Resistance=R  Inductance=10e-3  SetiL0=off  InitialCurrent=0  Capacitance=1e-6  Setx0=off  InitialVoltage=0  Measurements=None
  2 : powerlib/Elements/Series RLC Branch  LConnTagsString=__new0  RConnTagsString=__new0  BranchType=R  Resistance=R  Inductance=10e-3  SetiL0=off  InitialCurrent=0  Capacitance=1e-6  Setx0=off  InitialVoltage=0  Measurements=None
  3 : powerlib/Elements/Series RLC Branch  LConnTagsString=__new0  RConnTagsString=__new0  BranchType=R  Resistance=R  Inductance=10e-3  SetiL0=off  InitialCurrent=0  Capacitance=1e-6  Setx0=off  InitialVoltage=0  Measurements=None
  A : PMIOPort  Side=Left
  B : PMIOPort  Port=2  Side=Left
  C : PMIOPort  Port=3  Side=Left
  N : PMIOPort  Port=4  Side=Right
  connections:
  A/RConn1 -- 2/LConn1
  B/RConn1 -- 1/LConn1
  C/RConn1 -- 3/LConn1
  1/RConn1 -- 3/RConn1 -- N/RConn1 -- 2/RConn1

== system final_hybrid_system_load_variation/Load/Load4 ==
  1 : powerlib/Elements/Series RLC Branch  LConnTagsString=__new0  RConnTagsString=__new0  BranchType=R  Resistance=R  Inductance=10e-3  SetiL0=off  InitialCurrent=0  Capacitance=1e-6  Setx0=off  InitialVoltage=0  Measurements=None
  2 : powerlib/Elements/Series RLC Branch  LConnTagsString=__new0  RConnTagsString=__new0  BranchType=R  Resistance=R  Inductance=10e-3  SetiL0=off  InitialCurrent=0  Capacitance=1e-6  Setx0=off  InitialVoltage=0  Measurements=None
  3 : powerlib/Elements/Series RLC Branch  LConnTagsString=__new0  RConnTagsString=__new0  BranchType=R  Resistance=R  Inductance=10e-3  SetiL0=off  InitialCurrent=0  Capacitance=1e-6  Setx0=off  InitialVoltage=0  Measurements=None
  A : PMIOPort  Side=Left
  B : PMIOPort  Port=2  Side=Left
  C : PMIOPort  Port=3  Side=Left
  N : PMIOPort  Port=4  Side=Right
  connections:
  A/RConn1 -- 2/LConn1
  B/RConn1 -- 1/LConn1
  C/RConn1 -- 3/LConn1
  1/RConn1 -- 3/RConn1 -- N/RConn1 -- 2/RConn1

== system final_hybrid_system_load_variation/Load/Load5 ==
  1 : powerlib/Elements/Series RLC Branch  LConnTagsString=__new0  RConnTagsString=__new0  BranchType=R  Resistance=R  Inductance=10e-3  SetiL0=off  InitialCurrent=0  Capacitance=1e-6  Setx0=off  InitialVoltage=0  Measurements=None
  2 : powerlib/Elements/Series RLC Branch  LConnTagsString=__new0  RConnTagsString=__new0  BranchType=R  Resistance=R  Inductance=10e-3  SetiL0=off  InitialCurrent=0  Capacitance=1e-6  Setx0=off  InitialVoltage=0  Measurements=None
  3 : powerlib/Elements/Series RLC Branch  LConnTagsString=__new0  RConnTagsString=__new0  BranchType=R  Resistance=R  Inductance=10e-3  SetiL0=off  InitialCurrent=0  Capacitance=1e-6  Setx0=off  InitialVoltage=0  Measurements=None
  A : PMIOPort  Side=Left
  B : PMIOPort  Port=2  Side=Left
  C : PMIOPort  Port=3  Side=Left
  N : PMIOPort  Port=4  Side=Right
  connections:
  A/RConn1 -- 2/LConn1
  B/RConn1 -- 1/LConn1
  C/RConn1 -- 3/LConn1
  1/RConn1 -- 3/RConn1 -- N/RConn1 -- 2/RConn1

== system final_hybrid_system_load_variation/Load/Load6 ==
  1 : powerlib/Elements/Series RLC Branch  LConnTagsString=__new0  RConnTagsString=__new0  BranchType=R  Resistance=R  Inductance=10e-3  SetiL0=off  InitialCurrent=0  Capacitance=1e-6  Setx0=off  InitialVoltage=0  Measurements=None
  2 : powerlib/Elements/Series RLC Branch  LConnTagsString=__new0  RConnTagsString=__new0  BranchType=R  Resistance=R  Inductance=10e-3  SetiL0=off  InitialCurrent=0  Capacitance=1e-6  Setx0=off  InitialVoltage=0  Measurements=None
  3 : powerlib/Elements/Series RLC Branch  LConnTagsString=__new0  RConnTagsString=__new0  BranchType=R  Resistance=R  Inductance=10e-3  SetiL0=off  InitialCurrent=0  Capacitance=1e-6  Setx0=off  InitialVoltage=0  Measurements=None
  A : PMIOPort  Side=Left
  B : PMIOPort  Port=2  Side=Left
  C : PMIOPort  Port=3  Side=Left
  N : PMIOPort  Port=4  Side=Right
  connections:
  A/RConn1 -- 2/LConn1
  B/RConn1 -- 1/LConn1
  C/RConn1 -- 3/LConn1
  1/RConn1 -- 3/RConn1 -- N/RConn1 -- 2/RConn1

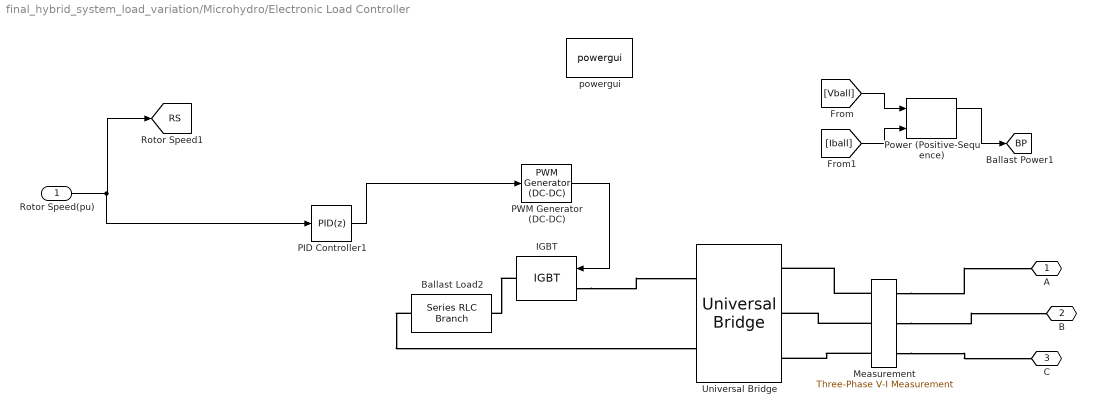
== system final_hybrid_system_load_variation/Microhydro/Electronic Load Controller ==
  Rotor Speed(pu) : Inport
  Ballast Load2 : powerlib/Elements/Series RLC Branch  LConnTagsString=__new0  RConnTagsString=__new0  BranchType=R  Resistance=10  Inductance=10e-3  SetiL0=off  InitialCurrent=0  Capacitance=1e-6  Setx0=off  InitialVoltage=0  Measurements=None
  IGBT : powerlib/Power Electronics/IGBT  Ron=0.001  Lon=0  Vf=1  Tf=1e-6  Tt=2e-6  IC=0  Rs=1e8  Cs=inf  Measurements=off
  Measurement : powerlib/Measurements/Three-Phase V-I Measurement  VoltageMeasurement=phase-to-ground  SetLabelV=on  LabelV=Vball  Vpu=off  VpuLL=off  CurrentMeasurement=yes  SetLabelI=on  LabelI=Iball  Ipu=off  Pbase=100e6  Vbase=500e3  OutputType=Complex  PhasorSimulation=off  PSBequivalent=0
  PID Controller1 : simulink/Continuous/PID Controller  Controller=PID  TimeDomain=Discrete-time  SampleTime=1e-6  IntegratorMethod=Forward Euler  FilterMethod=Forward Euler  Form=Ideal  UseFilter=off  ControllerParametersSource=internal  P=50  I=100  D=0.05  N=100  InitialConditionSource=internal  InitialConditionForIntegrator=0  InitialConditionForFilter=0  ExternalReset=none  ZeroCross=off  LimitOutput=on  UpperSaturationLimit=1  LowerSaturationLimit=0  LinearizeAsGain=on  AntiWindupMode=none  Kb=1  TrackingMode=off  Kt=1  PParamMin=[]  PParamMax=[]  IParamMin=[]  IParamMax=[]  DParamMin=[]  DParamMax=[]  NParamMin=[]  NParamMax=[]  KbParamMin=[]  KbParamMax=[]  KtParamMin=[]  KtParamMax=[]  POutMin=[]  POutMax=[]  IOutMin=[]  IOutMax=[]  DOutMin=[]  DOutMax=[]  NOutMin=[]  NOutMax=[]  KbOutMin=[]  KbOutMax=[]  KtOutMin=[]  KtOutMax=[]  IntegratorOutMin=[]  IntegratorOutMax=[]  FilterOutMin=[]  FilterOutMax=[]  SumOutMin=[]  SumOutMax=[]  SumI1OutMin=[]  SumI1OutMax=[]  SumI2OutMin=[]  SumI2OutMax=[]  SumI3OutMin=[]  SumI3OutMax=[]  SumDOutMin=[]  SumDOutMax=[]  SaturationOutMin=[]  SaturationOutMax=[]  IntegratorContinuousStateAttributes=''  IntegratorStateMustResolveToSignalObject=off  IntegratorRTWStateStorageClass=Auto  FilterContinuousStateAttributes=''  FilterStateMustResolveToSignalObject=off  FilterRTWStateStorageClass=Auto  DifferentiatorICPrevScaledInput=0  DifferentiatorOutMin=[]  DifferentiatorOutMax=[]  FilterDiffOutCoefMin=[]  FilterDiffOutCoefMax=[]  SumDenOutMin=[]  SumDenOutMax=[]  SumNumOutMin=[]  SumNumOutMax=[]  ReciprocalOutMin=[]  ReciprocalOutMax=[]  DivideOutMin=[]  DivideOutMax=[]  TunerSelectOption=Transfer Function Based (PID Tuner App)
  PWM Generator (DC-DC) : powerlib_meascontrol/Pulse & Signal Generators/PWM Generator (DC-DC)  Fsw=4000  Ts=1e-6
  Power (Positive-Sequence) : powerlib_meascontrol/Measurements/Power (Positive-Sequence)  Freq=50  Vinit=[0, 0]  Iinit=[0, 0]  Ts=0
      settings: SourceProductName=Simscape Power Systems  SourceProductBaseCode=PS
  Universal Bridge : powerlib/Power Electronics/Universal Bridge  Arms=3  SnubberResistance=1e6  SnubberCapacitance=10e-9  Device=Diodes  Ron=1e-3  Lon=0  ForwardVoltages="[  0  0  ]"  ForwardVoltage=0  GTOparameters=[ 10e-6 , 20e-6 ]  IGBTparameters=[ 1e-6 , 2e-6 ]  Measurements=None  Measurements_2=None  converterType=Rectifier
  powergui : powerlib/powergui  Priority=1  SimulationMode=Discrete  SampleTime=1e-6  frequency=50  Iterations=50  frequencyindice=0  Pbase=100e6  ErrMax=1e-4  UnitsV=kV  UnitsW=MW  buscounter=0  FunctionMessages=off  echomessages=off  EnableUseOfTLC=off  CurrentSourceSwitches=off  DisableSnubberDevices=off  DisableRonSwitches=off  DisableVfSwitches=off  DisplayEquations=off  SolverType=Tustin/Backward Euler (TBE)  Interpol=off  ExternalGateDelay=off  methode=off  Ts=100  x0status=zero  SPID=off  SwTol=0  HookPort=off  RestoreLinks=warning  ResistiveCurrentMeasurement=off  Frange=[0:2:500]  Ylog=off  Xlog=on  ShowGrid=off  save=off  variable=ZData  structure=Source_Current  ZoomFFT=on  StartTime=1.295  cycles=10  DisplayStyle=1  fundamental=50  FreqAxis=off  MaxFrequency=1000  frequencyindicesteady=1  RmsSteady=1  display=off
  A : PMIOPort  Side=Left
  B : PMIOPort  Port=2  Side=Left
  C : PMIOPort  Port=3  Side=Left
  tag scope: BP=global, RS=global
  wires:
  PID Controller1/1 -> PWM Generator (DC-DC)/1
  PWM Generator (DC-DC)/1 -> IGBT/1
  Rotor Speed(pu)/1 -> PID Controller1/1, [RS]
  Power (Positive-Sequence)/1 -> [BP]
  [Vball] -> Power (Positive-Sequence)/1
  [Iball] -> Power (Positive-Sequence)/2
  connections:
  Ballast Load2/RConn1 -- Universal Bridge/RConn2
  IGBT/LConn1 -- Universal Bridge/RConn1
  IGBT/RConn1 -- Ballast Load2/LConn1
  Measurement/RConn3 -- Universal Bridge/LConn3
  Measurement/RConn2 -- Universal Bridge/LConn2
  Measurement/RConn1 -- Universal Bridge/LConn1
  Measurement/LConn1 -- A/RConn1
  Measurement/LConn2 -- B/RConn1
  Measurement/LConn3 -- C/RConn1

== system final_hybrid_system_load_variation/PV-Syncronverter system/Signal Builder ==
  Demux : Demux  Tag=STV Demux  Outputs=1
  FromWs : FromWorkspace  Tag=STV FromWs  VariableName=tuvar  SampleTime=0
      SigBuilderData=|
      | common.afterFinalStr = 'Extrapolate'
      | common.sampleTime = 0
      | dataSet.timeRange = [0 10]
      | dataSet.name = 'Group 1'
      | sbobj.Groups.Name = 'Group 1'
      | sbobj.Groups.Signals.Name = 'Signal 1'
      | sbobj.Groups.Signals.XData = [0 1 3 4 10]
      | sbobj.Groups.Signals.YData = [1000 1000 -5 715 715]
  Signal 1 : Outport  Tag=STV Outport
  wires:
  Demux/1 -> Signal 1/1
  FromWs/1 -> Demux/1

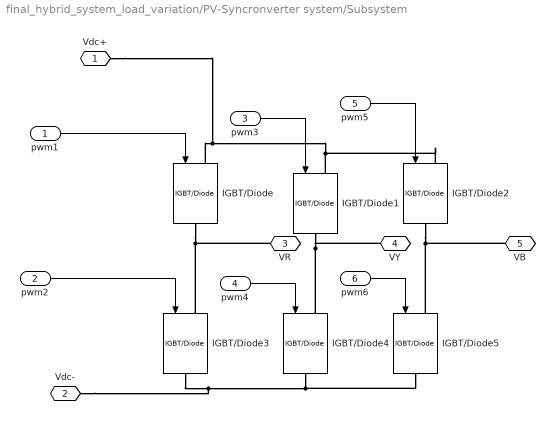
== system final_hybrid_system_load_variation/PV-Syncronverter system/Subsystem ==
  pwm1 : Inport
  pwm2 : Inport  Port=2
  pwm3 : Inport  Port=3
  pwm4 : Inport  Port=4
  pwm5 : Inport  Port=5
  pwm6 : Inport  Port=6
  IGBT/Diode{,1..5} (6 alike) : powerlib/Power Electronics/IGBT//Diode  Ron=1e-3  Rs=1e5  Cs=inf  Measurements=off
  Vdc+ : PMIOPort  Side=Left
  Vdc- : PMIOPort  Port=2  Side=Left
  VR : PMIOPort  Port=3  Side=Right
  VY : PMIOPort  Port=4  Side=Right
  VB : PMIOPort  Port=5  Side=Right
  wires:
  pwm4/1 -> IGBT/Diode4/1
  pwm1/1 -> IGBT/Diode/1
  pwm2/1 -> IGBT/Diode3/1
  pwm5/1 -> IGBT/Diode2/1
  pwm6/1 -> IGBT/Diode5/1
  pwm3/1 -> IGBT/Diode1/1
  connections:
  IGBT/Diode4/RConn1 -- IGBT/Diode5/RConn1 -- Vdc-/RConn1 -- IGBT/Diode3/RConn1
  IGBT/Diode1/RConn1 -- IGBT/Diode4/LConn1 -- VY/RConn1
  IGBT/Diode1/LConn1 -- IGBT/Diode2/LConn1 -- Vdc+/RConn1 -- IGBT/Diode/LConn1
  IGBT/Diode2/RConn1 -- IGBT/Diode5/LConn1 -- VB/RConn1
  IGBT/Diode/RConn1 -- IGBT/Diode3/LConn1 -- VR/RConn1

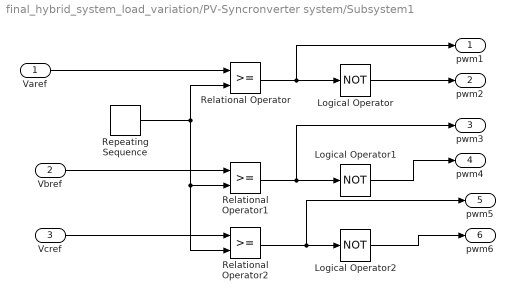
== system final_hybrid_system_load_variation/PV-Syncronverter system/Subsystem1 ==
  "Varef " : Inport
  Vbref : Inport  Port=2
  Vcref : Inport  Port=3
  Logical Operator : Logic  Operator=NOT  AllPortsSameDT=off  OutDataTypeStr=boolean
  Logical Operator1 : Logic  Operator=NOT  AllPortsSameDT=off  OutDataTypeStr=boolean
  Logical Operator2 : Logic  Operator=NOT  AllPortsSameDT=off  OutDataTypeStr=boolean
  Relational Operator : RelationalOperator  OutDataTypeStr=boolean  RndMeth=Simplest
  Relational Operator1 : RelationalOperator  OutDataTypeStr=boolean  RndMeth=Simplest
  Relational Operator2 : RelationalOperator  OutDataTypeStr=boolean  RndMeth=Simplest
  Repeating Sequence : simulink/Sources/Repeating Sequence  rep_seq_t=[0 0.00005 0.0001]  rep_seq_y=[-1 1 -1]
  pwm1 : Outport
  pwm2 : Outport  Port=2
  pwm3 : Outport  Port=3
  pwm4 : Outport  Port=4
  pwm5 : Outport  Port=5
  pwm6 : Outport  Port=6
  wires:
  Relational Operator/1 -> Logical Operator/1, pwm1/1
  Logical Operator/1 -> pwm2/1
  Vcref/1 -> Relational Operator2/1
  Logical Operator1/1 -> pwm4/1
  Relational Operator1/1 -> Logical Operator1/1, pwm3/1
  Relational Operator2/1 -> Logical Operator2/1, pwm5/1
  "Varef "/1 -> Relational Operator/1
  Repeating Sequence/1 -> Relational Operator1/2, Relational Operator2/2, Relational Operator/2
  Vbref/1 -> Relational Operator1/1
  Logical Operator2/1 -> pwm6/1

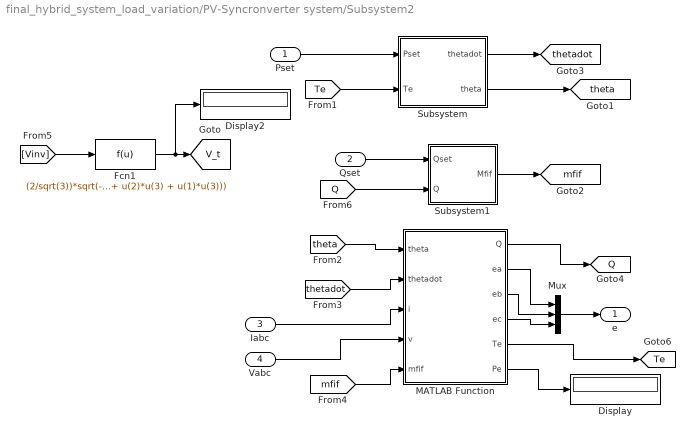
== system final_hybrid_system_load_variation/PV-Syncronverter system/Subsystem2 ==
  "Pset " : Inport
  Qset : Inport  Port=2
  "Iabc " : Inport  Port=3
  Vabc : Inport  Port=4
  Display : Display
  Display2 : Display
  Fcn1 : Fcn  Expr="(2/sqrt(3))*sqrt(-(u(1)*u(2)  + u(2)*u(3) + u(1)*u(3)))"
  MATLAB Function : MATLAB Function  TreatAsAtomicUnit=on
  Mux : Mux  Inputs=3
  Subsystem : Subsystem
  Subsystem1 : Subsystem
  e : Outport
  tag scope: Q=global, Te=global, V_t=global, mfif=global, theta=global, thetadot=global
  wires:
  "Pset "/1 -> Subsystem/1("Pset ")
  [Q] -> Subsystem1/2(Q)
  Subsystem1/1(Mfif) -> [mfif]
  Subsystem/1("thetadot ") -> [thetadot]
  Subsystem/2(theta) -> [theta]
  [Te] -> Subsystem/2(Te)
  [thetadot] -> MATLAB Function/2(thetadot)
  "Iabc "/1 -> MATLAB Function/3(i)
  [mfif] -> MATLAB Function/5(mfif)
  MATLAB Function/1(Q) -> [Q]
  MATLAB Function/5(Te) -> [Te]
  MATLAB Function/2(ea) -> Mux/1
  MATLAB Function/3(eb) -> Mux/2
  MATLAB Function/4(ec) -> Mux/3
  Mux/1 -> e/1
  [theta] -> MATLAB Function/1(theta)
  [Vinv] -> Fcn1/1
  Fcn1/1 -> Display2/1, [V_t]
  MATLAB Function/6(Pe) -> Display/1
  Vabc/1 -> MATLAB Function/4(v)
  Qset/1 -> Subsystem1/1(Qset)

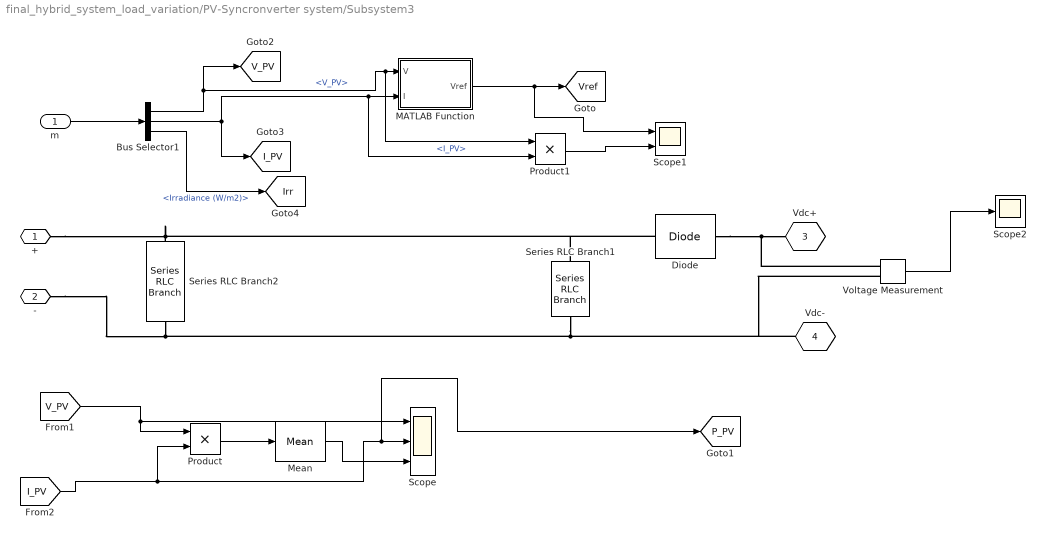
== system final_hybrid_system_load_variation/PV-Syncronverter system/Subsystem3 ==
  m : Inport
  Bus Selector1 : BusSelector  OutputSignals=V_PV,I_PV,Irradiance (W/m2)
  Diode : powerlib/Power Electronics/Diode  Ron=0.001  Lon=0  Vf=0.8  IC=0  UseSnubber=0  Rs=500  Cs=250e-9  Measurements=off
  MATLAB Function : MATLAB Function  TreatAsAtomicUnit=on
  Mean : powerlib_meascontrol/Measurements/Mean  Freq=50  Vinit=0  Ts=0
  Product : Product
  Product1 : Product
  Scope : Scope  NumInputPorts=3
  Scope1 : Scope  NumInputPorts=2
  Scope2 : Scope
  Series RLC Branch1 : powerlib/Elements/Series RLC Branch  LConnTagsString=__new0  RConnTagsString=__new0  BranchType=RC  Resistance=1e-3  Inductance=1e-3  SetiL0=off  InitialCurrent=0  Capacitance=1000e-6  Setx0=off  InitialVoltage=0  Measurements=None
  Series RLC Branch2 : powerlib/Elements/Series RLC Branch  LConnTagsString=__new0  RConnTagsString=__new0  BranchType=RC  Resistance=1e-3  Inductance=1e-3  SetiL0=off  InitialCurrent=0  Capacitance=1000e-6  Setx0=off  InitialVoltage=0  Measurements=None
  Voltage Measurement : powerlib/Measurements/Voltage Measurement  PhasorSimulation=off  OutputType=Complex  PSBequivalent=0
  + : PMIOPort  Side=Left
  - : PMIOPort  Port=2  Side=Left
  Vdc+ : PMIOPort  Tag=PMCPort  Port=3  Side=Right
  Vdc- : PMIOPort  Tag=PMCPort  Port=4  Side=Right
  tag scope: I_PV=global, Irr=global, P_PV=global, V_PV=global, Vref=global
  wires:
  Bus Selector1/1 -> [V_PV], Product1/1, MATLAB Function/1(V)  "<V_PV>"
  m/1 -> Bus Selector1/1
  Bus Selector1/2 -> [I_PV], Product1/2, MATLAB Function/2(I)  "<I_PV>"
  [V_PV] -> Scope/1, Product/1
  Product/1 -> Mean/1
  MATLAB Function/1(Vref) -> Scope1/1, [Vref]
  Product1/1 -> Scope1/2
  [I_PV] -> [P_PV], Scope/2, Product/2
  Mean/1 -> Scope/3
  Bus Selector1/3 -> [Irr]  "<Irradiance (W/m2)>"
  Voltage Measurement/1 -> Scope2/1
  connections:
  Voltage Measurement/LConn2 -- Vdc-/RConn1 -- Series RLC Branch1/RConn1 -- -/RConn1 -- Series RLC Branch2/RConn1
  Series RLC Branch2/LConn1 -- Diode/LConn1 -- Series RLC Branch1/LConn1 -- +/RConn1
  Diode/RConn1 -- Voltage Measurement/LConn1 -- Vdc+/RConn1

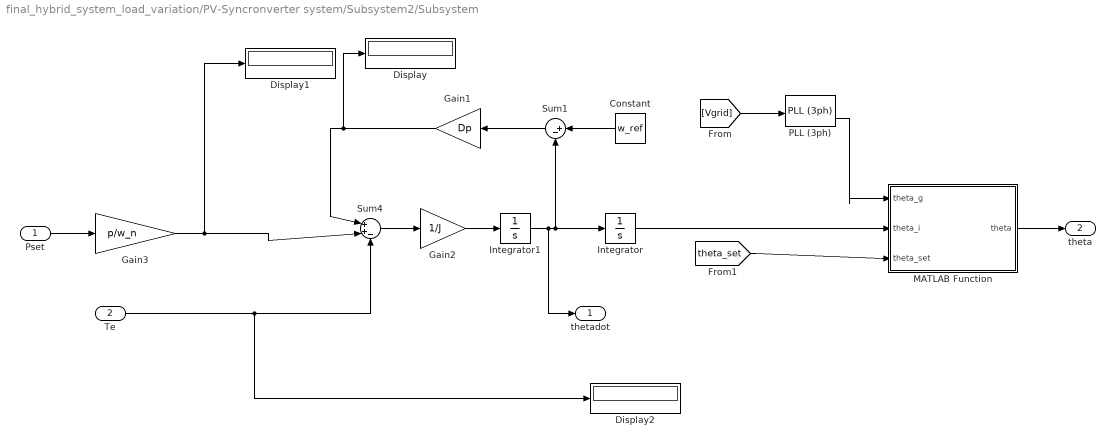
== system final_hybrid_system_load_variation/PV-Syncronverter system/Subsystem2/Subsystem ==
  "Pset " : Inport
  Te : Inport  Port=2
  Constant : Constant  Value=w_ref
  Display : Display
  Display1 : Display
  Display2 : Display
  Gain1 : Gain  Gain=Dp
  Gain2 : Gain  Gain=1/J
  Gain3 : Gain  Gain=p/w_n
  Integrator : Integrator
  Integrator1 : Integrator  InitialCondition=w_n
  MATLAB Function : MATLAB Function  TreatAsAtomicUnit=on
  PLL (3ph) : powerlib_meascontrol/PLL/PLL (3ph)  Fmin=45  Par_Init=[0, 50]  ParK=[150, 4000,0]  TcD=1e-6  MaxRateChangeFreq=12  FilterCutOffFreq=25  Ts=Ts  AGC=on
  Sum1 : Sum  Inputs=|+-
  Sum4 : Sum  Inputs=|++-
  "thetadot " : Outport
  theta : Outport  Port=2
  wires:
  Sum1/1 -> Gain1/1
  Constant/1 -> Sum1/1
  Gain2/1 -> Integrator1/1
  "Pset "/1 -> Gain3/1
  Sum4/1 -> Gain2/1
  Gain1/1 -> Display/1, Sum4/1
  Integrator1/1 -> "thetadot "/1, Integrator/1, Sum1/2
  Gain3/1 -> Display1/1, Sum4/2
  Te/1 -> Sum4/3, Display2/1
  [Vgrid] -> PLL (3ph)/1
  MATLAB Function/1(theta) -> theta/1
  Integrator/1 -> MATLAB Function/2(theta_i)
  PLL (3ph)/2 -> MATLAB Function/1(theta_g)
  [theta_set] -> MATLAB Function/3(theta_set)

== system final_hybrid_system_load_variation/PV-Syncronverter system/Subsystem2/Subsystem1 ==
  note: Mfif
  Qset : Inport
  Q : Inport  Port=2
  Constant : Constant  Value=400*sqrt(2/3)
  Display : Display
  Display1 : Display
  Display2 : Display
  Gain3 : Gain  Gain=1/K
  Gain6 : Gain  Gain=Dq
  Integrator1 : Integrator
  Sum1 : Sum  Inputs=|+-
  Sum2 : Sum  Inputs=|-++
  Mfif : Outport
  wires:
  Gain6/1 -> Sum2/3
  Qset/1 -> Sum2/2
  Sum2/1 -> Display2/1, Gain3/1
  Integrator1/1 -> Display/1, Mfif/1
  Q/1 -> Sum2/1
  Gain3/1 -> Integrator1/1
  [V_t] -> Sum1/2
  Sum1/1 -> Display1/1, Gain6/1
  Constant/1 -> Sum1/1

== matlab function final_hybrid_system_load_variation/PV-Syncronverter system/Subsystem3/MATLAB Function ==
  data: V input; Vref output; I input
function Vref = RefGen(V,I)
Vrefmax = 900;
Vrefmin = 0;
Vrefinit = 750;
deltaVref = 1;
persistent Vold Pold Vrefold;

dataType = 'double';
if isempty(Vold)
    Vold = 0;
    Pold = 0;
    Vrefold = Vrefinit;
end 

P = V*I;
dV = V-Vold;
dP = P-Pold;

if dP ~= 0
    if dP<0
        if dV < 0
            Vref = Vrefold+deltaVref;
        else 
            Vref = Vrefold -deltaVref;
        end 
    else 
        if dV<0
            Vref = Vrefold -deltaVref;
        else
            Vref = Vrefold + deltaVref;
        end
    end
else Vref = Vrefold;
end

if Vref >= Vrefmax | Vref<= Vrefmin
    Vref = Vrefold;
end

Vrefold = Vref;
Vold = V;
Pold = P;

== matlab function final_hybrid_system_load_variation/PV-Syncronverter system/Subsystem2/MATLAB Function ==
  data: theta input; Q output; thetadot input; i input; v input; mfif input; ea output; eb output; ec output; Te output; Pe output
function [Q,ea,eb,ec,Te,Pe] = syncronverter(theta,thetadot,i,v,mfif)
p=1;
w_n = 2*pi*50;
ea = thetadot*mfif*sin(theta);
eb = thetadot*mfif*sin(theta-120*pi/180);
ec = thetadot*mfif*sin(theta-240*pi/180);
Te = p*mfif*(i(1)*sin(theta) + i(2)*sin(theta-120*pi/180) + i(3)*sin(theta-240*pi/180));
Pe = v(1)*i(1) + v(2)*i(2) + v(3)*i(3);

Q = -thetadot*mfif*(i(1)*cos(theta) + i(2)*cos(theta - 120*pi/180) + i(3)*cos(theta - 240*pi/180));

== matlab function final_hybrid_system_load_variation/PV-Syncronverter system/Subsystem2/Subsystem/MATLAB Function ==
  data: theta_g input; theta output; theta_i input; theta_set input
function theta = fcn(theta_g, theta_i,theta_set)
if theta_i > 100
    theta = theta_g - theta_set*pi/180;
else 
    theta = theta_i;
end
end
